simulink model "ass3q2"  (R2025a)
settings: Solver=VariableStepAuto  StartTime=0.0  StopTime=1000  RelTol=1e-3
values from neighbouring files (symbols this model uses):
  D = 20 / ( 2 * pi)    (= 3.18309886184)    [assignement_3_simulink_q1.m]    (also in ecse563_part1c_model.m)
  M = length(nfrom)    [admittance.m]    (also in assignement_3_simulink_q1.m = 111.41; ecse563_part1c_model.m = 111.4; nrpf.m = zeros(nb, nb))
  R1 = 0.0060 * 2 * pi    (= 0.0376991118431)    [assignement_3_simulink_q1.m]
  R2 = 0.0120 * 2 * pi    (= 0.0753982236862)    [assignement_3_simulink_q1.m]
  Tch1 = 3    [assignement_3_simulink_q1.m]
  Tch2 = 8    [assignement_3_simulink_q1.m]
  Tg1 = 0.25    [assignement_3_simulink_q1.m]
  Tg2 = 0.50    (= 0.5)    [assignement_3_simulink_q1.m]
undefined symbols (not defined in the file or in its folder): K
settings Model: Creator=aliseifeldin  LastModifiedBy=aliseifeldin

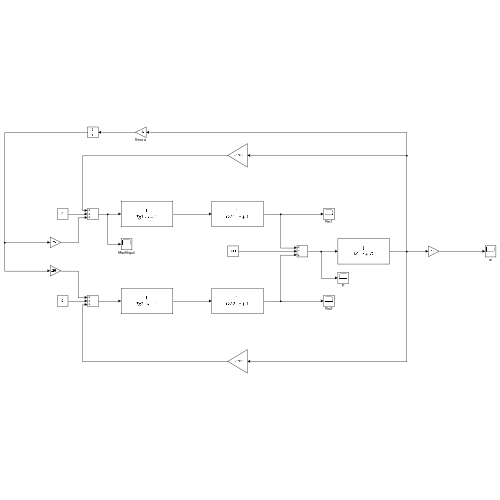
[thumbnail: Simulink's stored preview of the top-level diagram]
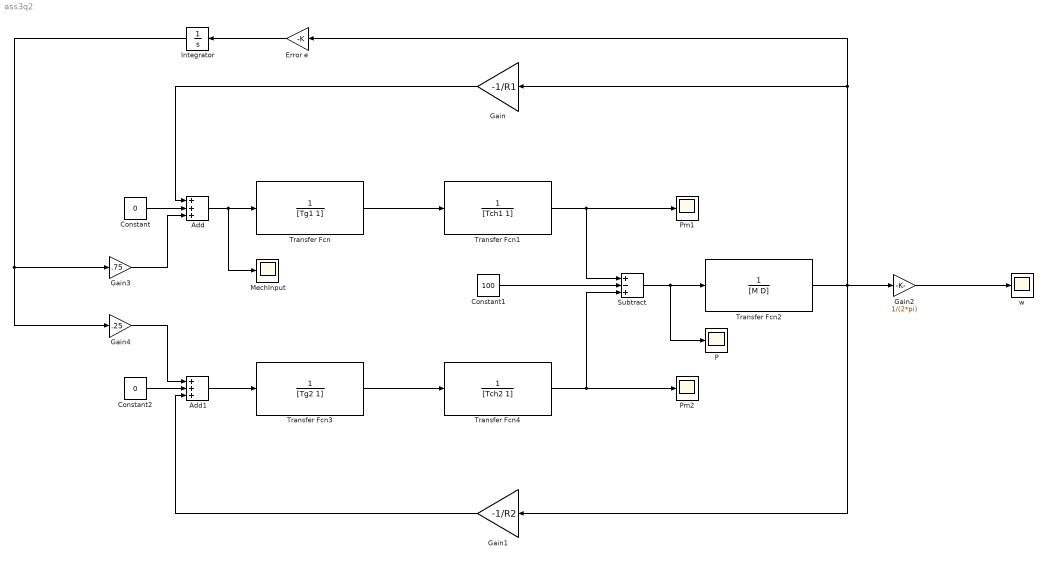
== system ass3q2 ==
  Add : Sum  Inputs=+++
  Add1 : Sum  Inputs=+++
  Constant : Constant  Value=0
  Constant1 : Constant  Value=100
  Constant2 : Constant  Value=0
  Error e : Gain  Gain=-K
  Gain : Gain  Gain=-1/R1
  Gain1 : Gain  Gain=-1/R2
  Gain2 : Gain  Gain=1/(2*pi)
  Gain3 : Gain  Gain=.75
  Gain4 : Gain  Gain=.25
  Integrator : Integrator
  MechInput : Scope
      settings: ActiveDisplayYMinimum=-10.410800299026624  ActiveDisplayYMaximum=93.697202691239625  DataLoggingVariableName=Pm1Scope1
  P : Scope
      settings: ActiveDisplayYMinimum=-0.041590845623852131  ActiveDisplayYMaximum=-0.0047623872769294792  DataLoggingVariableName=PScope
  Pm1 : Scope
      settings: ActiveDisplayYMinimum=-10.410800299026624  ActiveDisplayYMaximum=93.697202691239625  DataLoggingVariableName=Pm1Scope
  Pm2 : Scope
      settings: ActiveDisplayYMinimum=-3.9741691062345192  ActiveDisplayYMaximum=35.767521956110684  DataLoggingVariableName=Pm2Scope
  Subtract : Sum  Inputs=+-+
  Transfer Fcn : TransferFcn  Denominator=[Tg1 1]
  Transfer Fcn1 : TransferFcn  Denominator=[Tch1 1]
  Transfer Fcn2 : TransferFcn  Denominator=[M D]
  Transfer Fcn3 : TransferFcn  Denominator=[Tg2 1]
  Transfer Fcn4 : TransferFcn  Denominator=[Tch2 1]
  w : Scope
      settings: ActiveDisplayYMinimum=-3.9848441193370876  ActiveDisplayYMaximum=0.44276045770412076  DataLoggingVariableName=wScope
  wires:
  Transfer Fcn/1 -> Transfer Fcn1/1
  Subtract/1 -> P/1, Transfer Fcn2/1
  Transfer Fcn1/1 -> Pm1/1, Subtract/1
  Transfer Fcn2/1 -> Gain2/1, Error e/1, Gain/1, Gain1/1
  Gain/1 -> Add/1
  Add/1 -> MechInput/1, Transfer Fcn/1
  Constant/1 -> Add/2
  Constant1/1 -> Subtract/2
  Transfer Fcn3/1 -> Transfer Fcn4/1
  Add1/1 -> Transfer Fcn3/1
  Constant2/1 -> Add1/2
  Transfer Fcn4/1 -> Pm2/1, Subtract/3
  Gain2/1 -> w/1
  Error e/1 -> Integrator/1
  Gain1/1 -> Add1/3
  Gain4/1 -> Add1/1
  Gain3/1 -> Add/3
  Integrator/1 -> Gain4/1, Gain3/1
